simulink model "SEA_SMC_DoB"  (R2020a)
settings: Solver=FixedStepAuto  StartTime=0.0  StopTime=10.0  FixedStep=1e-4  RelTol=1e-3
undefined symbols (not defined in the file): A, B, C, D, SEA
libraries: simulink x6, cstblocks x4, cjt_library_models x1
settings Model: LastModifiedBy=Erim Can Ozcinar

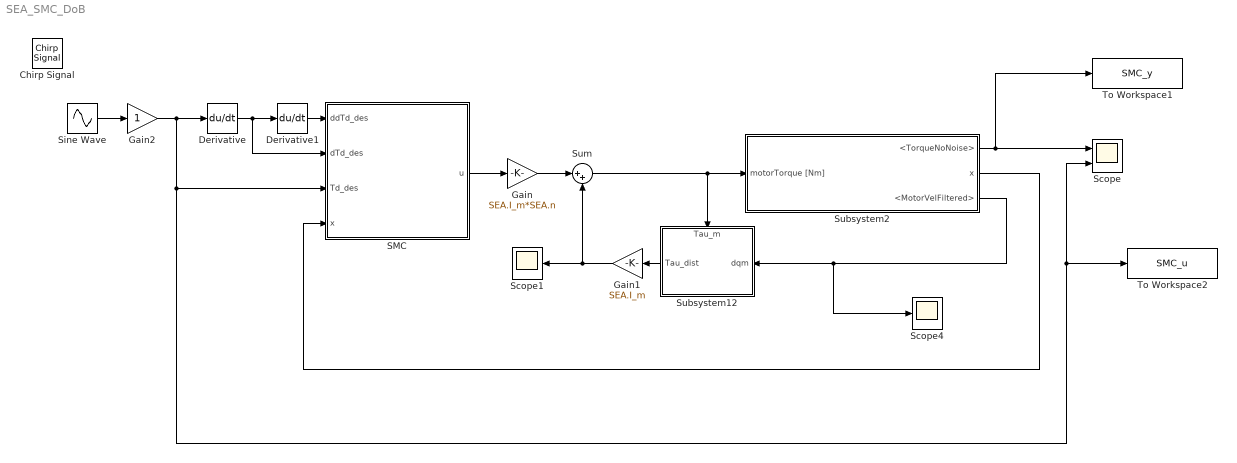
== system SEA_SMC_DoB ==
  Chirp Signal : simulink/Sources/Chirp Signal  f1=0.1  T=10  f2=25
  Derivative : Derivative
  Derivative1 : Derivative
  Gain : Gain  Gain=SEA.I_m*SEA.n
  Gain1 : Gain  Gain=SEA.I_m
  Gain2 : Gain
  SMC : MATLAB Function  TreatAsAtomicUnit=on
  Scope : Scope  NumInputPorts=2
  Scope1 : Scope
  Scope4 : Scope
  Sine Wave : Sin  SampleTime=0
  Subsystem12 : Subsystem
      settings: PortSchema="{\"entries\":[{\"content\":{\"sides\":[{\"content\":{\"connectorIds\":[\"In1\"]},\"type\":\"ConnectorPlacement.EquallySpacedRectSide\",\"uuid\":\"0907aefd-0f6e-4178-ae67-82d4302ffa8c\"},{\"content\":{\"connectorIds\":[\"Out1\"],\"side\":\"RIGHT\"},\"type\":\"ConnectorPlacement.EquallySpacedRectSide\",\"uuid\":\"771a5b93-7111-4ff8-830e-f982bc5484c0\"},{\"content\":{\"connectorIds\":[\"In2\"],\"side\":\"TOP\"},\"type\":\"ConnectorPlacement.EquallySpacedRectSide\",\"uuid\":\"5e11dad7-4fb7-439c-966f-d215f4d3795f\"}]},\"type\":\"ConnectorPlacement.EquallySpacedConnector\",\"uuid\":\"deab52ae-9dbd-41da-8fe4-7a69fd8df393\"}],\"packageUris\":[\"http://schema.mathworks.com/mf0/Connector/19700101\"],\"version\":\"1.0\"}"
  Subsystem2 : Subsystem
  Sum : Sum  Inputs=|++
  To Workspace1 : ToWorkspace  VariableName=SMC_y  SampleTime=-1
      settings: Save2DSignal=2-D array (concatenate along first dimension)
  To Workspace2 : ToWorkspace  VariableName=SMC_u  SampleTime=-1
      settings: Save2DSignal=2-D array (concatenate along first dimension)
  wires:
  Subsystem2/3(<MotorVelFiltered>) -> Scope4/1, Subsystem12/1(dqm)
  Sum/1 -> Subsystem2/1(motorTorque [Nm]), Subsystem12/2(Tau_m)
  Subsystem2/2(x) -> SMC/4(x)
  Subsystem12/1(Tau_dist) -> Gain1/1
  Gain1/1 -> Sum/2, Scope1/1
  Gain/1 -> Sum/1
  SMC/1(u) -> Gain/1
  Subsystem2/1(<TorqueNoNoise>) -> To Workspace1/1, Scope/1
  Derivative1/1 -> SMC/1(ddTd_des)
  Derivative/1 -> SMC/2(dTd_des), Derivative1/1
  Gain2/1 -> SMC/3(Td_des), Scope/2, To Workspace2/1, Derivative/1
  Sine Wave/1 -> Gain2/1

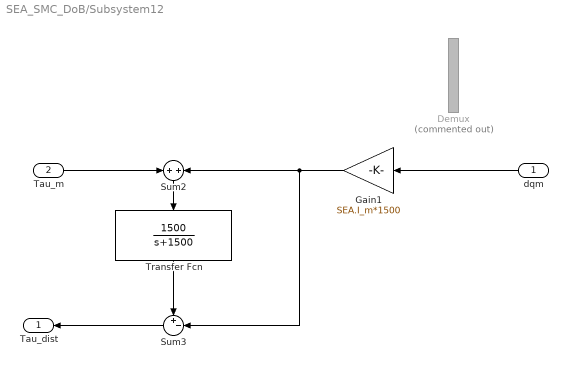
== system SEA_SMC_DoB/Subsystem12 ==
  dqm : Inport
  Tau_m : Inport  Port=2
  Demux : Demux  Commented=on  Outputs=3
  Gain1 : Gain  Gain=SEA.I_m*1500
  Sum2 : Sum  Inputs=+|+
  Sum3 : Sum  Inputs=+-|
  Transfer Fcn : TransferFcn  Numerator=[1500]  Denominator=[1 1500]
  Tau_dist : Outport
  wires:
  Gain1/1 -> Sum3/2, Sum2/2
  Sum3/1 -> Tau_dist/1
  Transfer Fcn/1 -> Sum3/1
  Tau_m/1 -> Sum2/1
  Sum2/1 -> Transfer Fcn/1
  dqm/1 -> Gain1/1

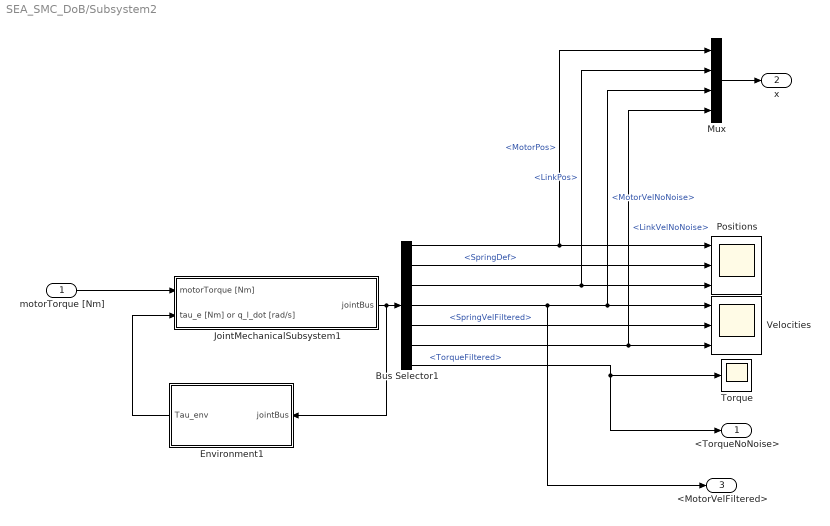
== system SEA_SMC_DoB/Subsystem2 ==
  motorTorque [Nm] : Inport
  Bus Selector1 : BusSelector  OutputSignals=MotorPos,SpringDef,LinkPos,MotorVelNoNoise,SpringVelFiltered,LinkVelNoNoise,TorqueFiltered
  Environment1 : Subsystem
  JointMechanicalSubsystem1 : Subsystem  AncestorBlock=cjt_library_models/Joint models/JointMechanicalSubsystem  mask(jointMechanicalSubsystem){jointObj=SEA, fc_vel=1000, fc_torque=1000, input_delay=0, output_delay=0, quantize=on, quantize_bits=19, input_noise_enabled=off, output_noise_enabled=off, var_u=0.000021, var_y=1e-10}
      mask prompts: jointObj "Joint Object"; fc_vel "Velocity filter cut-off frequency [Hz]"; fc_torque "Torque filter cut-off frequency [Hz]"; input_delay "Motor torque input delay (num samples of Ts)"; output_delay "Output delay (num samples of Ts)"; quantize "Quantize measurements"; quantize_bits "Quantization bits"; input_noise_enabled "Enable input noise"; output_noise_enabled "Enable measurement noise"; var_u "Input noise variance"; var_y "Measurement noise variance"
      mask help:
      | This block implements the mechanical dynamics of the actuator.
      |
      | For more information, see the > Help <.
      mask init:
      | % Get linear dynamics matrices
      | [A, B, C, D, I, R, K] = jointObj.getDynamicsMatrices();
      | 
      | % Build B matrix for nonlinear components
      | B_nonlinear = [zeros([size(B,1)-size(I,1),1]); 1./diag(I)];
      | 
      | % Get other properties
      | Ts      = jointObj.Ts;
      | Ts_elec = jointObj.Ts_elec;
      | k_b     = jointObj.k_b;
      | k_t     = jointObj.k_t;
      | n       = jointObj.n;
      | d_gl    = jointObj.d_gl;
      | 
      | % Handle MATLAB function block
      | handleMatlabFunctionBlock(gcb, jointObj);
      | 
      | % If input delay is enabled, set the flag to 1
      | input_delay_enable = 0;
      | if (input_delay > 0)
      |     input_delay_enable = 1;
      | end
      | 
      | % If noise is disabled, overwrite the given variances
      | if (input_noise_enabled == 0)
      |     var_u = 0;
      | end
      | if (output_noise_enabled == 0)
      | 	var_y = 0;
      | end
      mask Help:
      | This block implements the mechanical dynamics of the actuator. Depending on the configuration in which the joint class was built, its dynamics are given by one of the variants provided by the toolbox (see model/linear/). If provided, the linear dynamics are enhanced with nonlinear components.
      | 
      | <b>Inputs</b>
      | <b>motorTorque</b>: Electromechanical motor torque provided on the rotor. An input delay can be added to this input (e.g. due to communication delays or a very simplified representation of electrical dynamics).
      | <b>tau_e or q_l_dot</b>: External interaction torque. Depending on the selected linear dynamics model of the joint, this is either the external torque acting on the load or the imposed load velocity (for fixed-output models).
      | 
      | <b>Outputs</b>
      | <b>jointBus</b>: The various variables and their measurements, with optional delays/noise/quantisation etc. For most outputs, several instances exist. Output variables ending in "NoNoise" denote physical quantities, without noise, filtering, or delays. All other variables are affected by noise and delays (if enabled). Lastly, variables ending in "Filtered" are also low-pass filtered, with cut-off frequency set in the mask.
      | 
      | <b>An important note with regards to output variables associated with torque.</b>
      | The "Torque" and "TorqueFiltered" are computed in the way torque is usually sensed by the control system; deflection times spring constant, i.e. only the stiffness contribution is considered, as usually the internal damping of the used flexible element (parameter d_gl) is very small. Hence, TorqueFiltered is used by the toolbox controllers as well.
      | However, as noted before, "TorqueNoNoise" denotes the physical quantity. This means that it includes the torque produced by internal damping of the elastic element (parameter d_gl).
      mask Callback quantize: toggleMaskFields(gcbh, 'quantize', 'quantize_bits');
      mask Callback input_noise_enabled: toggleMaskFields(gcbh, 'input_noise_enabled', 'var_u');
      mask Callback output_noise_enabled: toggleMaskFields(gcbh, 'output_noise_enabled', 'var_y');
  Mux : Mux
  Positions : Scope  NumInputPorts=3
  Torque : Scope
  Velocities : Scope  NumInputPorts=3
  <TorqueNoNoise> : Outport
  x : Outport  Port=2
  <MotorVelFiltered> : Outport  Port=3
  wires:
  JointMechanicalSubsystem1/1(jointBus) -> Environment1/1(jointBus), Bus Selector1/1
  Mux/1 -> x/1
  Environment1/1(Tau_env) -> JointMechanicalSubsystem1/2(tau_e [Nm] or q_l_dot [rad/s])
  Bus Selector1/1 -> Mux/1, Positions/1  "<MotorPos>"
  Bus Selector1/2 -> Positions/2  "<SpringDef>"
  Bus Selector1/3 -> Mux/2, Positions/3  "<LinkPos>"
  Bus Selector1/4 -> <MotorVelFiltered>/1, Mux/3, Velocities/1  "<MotorVelNoNoise>"
  Bus Selector1/5 -> Velocities/2  "<SpringVelFiltered>"
  Bus Selector1/6 -> Mux/4, Velocities/3  "<LinkVelNoNoise>"
  Bus Selector1/7 -> <TorqueNoNoise>/1, Torque/1  "<TorqueFiltered>"
  motorTorque [Nm]/1 -> JointMechanicalSubsystem1/1(motorTorque [Nm])

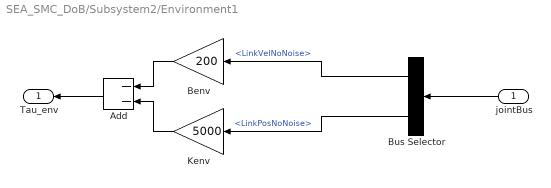
== system SEA_SMC_DoB/Subsystem2/Environment1 ==
  jointBus : Inport
  Add : Sum  Inputs=--
  Benv : Gain  Gain=200
  Bus Selector : BusSelector  OutputSignals=LinkVelNoNoise,LinkPosNoNoise
  Kenv : Gain  Gain=5000
  Tau_env : Outport
  wires:
  Kenv/1 -> Add/2
  Benv/1 -> Add/1
  Add/1 -> Tau_env/1
  Bus Selector/1 -> Benv/1  "<LinkVelNoNoise>"
  Bus Selector/2 -> Kenv/1  "<LinkPosNoNoise>"
  jointBus/1 -> Bus Selector/1

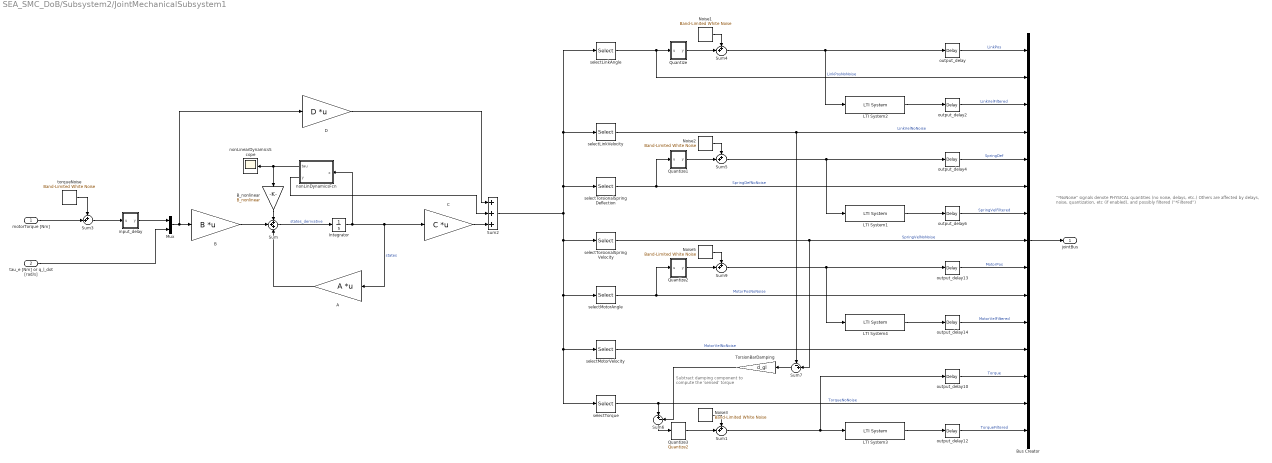
== system SEA_SMC_DoB/Subsystem2/JointMechanicalSubsystem1 ==
  note: "*NoNoise" signals denote PHYSICAL quantities (no noise, delays, etc.)
      | Others are affected by delays, noise, quantization, etc (if enabled), and possibly filtered ("*Filtered")
  note: Subtract damping component to
      | compute the 'sensed' torque
  motorTorque [Nm] : Inport
  tau_e [Nm] or q_l_dot [rad/s] : Inport  Port=2
  A : Gain  Gain=A  Multiplication=Matrix(K*u)
  B : Gain  Gain=B  Multiplication=Matrix(K*u)
  B_nonlinear : Gain  Gain=B_nonlinear
  Bus Creator : BusCreator  Inputs=15
  C : Gain  Gain=C  Multiplication=Matrix(K*u)
  D : Gain  Gain=D  Multiplication=Matrix(K*u)
  Integrator : Integrator
  LTI System1 : cstblocks/LTI System  sys=c2d(tf([2*pi*fc_vel 0], [1 2*pi*fc_vel]), Ts, 'tustin')  IC=[]
  LTI System2 : cstblocks/LTI System  sys=c2d(tf([2*pi*fc_vel 0], [1 2*pi*fc_vel]), Ts, 'tustin')  IC=[]
  LTI System3 : cstblocks/LTI System  sys=c2d(tf([2*pi*fc_torque], [1 2*pi*fc_torque]), Ts, 'tustin')  IC=[]
  LTI System4 : cstblocks/LTI System  sys=c2d(tf([2*pi*fc_vel 0], [1 2*pi*fc_vel]), Ts, 'tustin')  IC=[]
  Mux : Mux  Inputs=2
  Noise1 : simulink/Sources/Band-Limited White Noise  Cov=var_y * Ts  Ts=Ts  seed=[3846513]
  Noise2 : simulink/Sources/Band-Limited White Noise  Cov=var_y * Ts  Ts=Ts  seed=[11563454]
  Noise3 : simulink/Sources/Band-Limited White Noise  Cov=sqrt(2) * var_y * Ts % sqrt(2) accounts for subtracting two encoders  Ts=Ts  seed=[960834]
  Noise5 : simulink/Sources/Band-Limited White Noise  Cov=var_y * Ts  Ts=Ts  seed=[24326]
  Quantize : Subsystem
  Quantize1 : Subsystem
  Quantize2 : Subsystem
  Quantize3 : cjt_library_models/Joint models/JointMechanicalSubsystem/Quantize2  SystemSampleTime=-1  Latency=0  AutoFrameSizeCalculation=off
  Sum : Sum  Inputs=+++
  Sum{1,3..5,9} (5 alike) : Sum  Inputs=++|
  Sum2 : Sum  Inputs=+++
  Sum6 : Sum  Inputs=|+-
  Sum7 : Sum  Inputs=-+|
  TorsionBarDamping : Gain  Gain=d_gl
  input_delay : Subsystem
  nonLinDynamicsFcn : MATLAB Function  TreatAsAtomicUnit=on
  nonLinearDynamicsScope : Scope
  output_delay{,2,4,6,10,12..14} (8 alike) : TransportDelay  DelayTime=output_delay * jointObj.Ts
  selectLinkAngle : Selector  NumberOfDimensions=2  InputPortWidth=3  IndexOptions=Index vector (dialog),Select all  Indices=3,1  OutputSizes=1,1
  selectLinkVelocity : Selector  NumberOfDimensions=2  InputPortWidth=3  IndexOptions=Index vector (dialog),Select all  Indices=6,1  OutputSizes=1,1
  selectMotorAngle : Selector  NumberOfDimensions=2  InputPortWidth=3  IndexOptions=Index vector (dialog),Select all  Indices=1,1  OutputSizes=1,1
  selectMotorVelocity : Selector  NumberOfDimensions=2  InputPortWidth=3  IndexOptions=Index vector (dialog),Select all  Indices=4,1  OutputSizes=1,1
  selectTorque : Selector  NumberOfDimensions=2  InputPortWidth=3  IndexOptions=Index vector (dialog),Select all  Indices=7,1  OutputSizes=1,1
  selectTorsionalSpringDeflection : Selector  NumberOfDimensions=2  InputPortWidth=3  IndexOptions=Index vector (dialog),Select all  Indices=2,1  OutputSizes=1,1
  selectTorsionalSpringVelocity : Selector  NumberOfDimensions=2  InputPortWidth=3  IndexOptions=Index vector (dialog),Select all  Indices=5,1  OutputSizes=1,1
  torqueNoise : simulink/Sources/Band-Limited White Noise  Cov=var_u * Ts  Ts=Ts  seed=[2435345645]
  jointBus : Outport
  wires:
  Sum6/1 -> Quantize3/1
  Noise3/1 -> Sum1/1
  Quantize3/1 -> Sum1/2
  Sum7/1 -> TorsionBarDamping/1
  TorsionBarDamping/1 -> Sum6/2
  C/1 -> Sum2/3
  D/1 -> Sum2/1
  Quantize2/1(y) -> Sum9/2
  Quantize1/1(y) -> Sum5/2
  Quantize/1(y) -> Sum4/2
  Sum1/1 -> LTI System3/1, output_delay10/1
  LTI System3/1 -> output_delay12/1
  tau_e [Nm] or q_l_dot [rad/s]/1 -> Mux/2
  Mux/1 -> B/1, D/1
  Sum9/1 -> output_delay13/1, LTI System4/1
  output_delay14/1 -> Bus Creator/11  "MotorVelFiltered"
  output_delay13/1 -> Bus Creator/9  "MotorPos"
  LTI System4/1 -> output_delay14/1
  Noise5/1 -> Sum9/1
  output_delay12/1 -> Bus Creator/15  "TorqueFiltered"
  selectTorque/1 -> Bus Creator/14, Sum6/1  "TorqueNoNoise"
  output_delay10/1 -> Bus Creator/13  "Torque"
  selectMotorVelocity/1 -> Bus Creator/12  "MotorVelNoNoise"
  selectMotorAngle/1 -> Bus Creator/10, Quantize2/1(u)  "MotorPosNoNoise"
  selectTorsionalSpringVelocity/1 -> Sum7/2, Bus Creator/8  "SpringVelNoNoise"
  output_delay6/1 -> Bus Creator/7  "SpringVelFiltered"
  selectTorsionalSpringDeflection/1 -> Bus Creator/6, Quantize1/1(u)  "SpringDefNoNoise"
  output_delay4/1 -> Bus Creator/5  "SpringDef"
  selectLinkVelocity/1 -> Sum7/1, Bus Creator/4  "LinkVelNoNoise"
  output_delay2/1 -> Bus Creator/3  "LinkVelFiltered"
  selectLinkAngle/1 -> Bus Creator/2, Quantize/1(u)  "LinkPosNoNoise"
  output_delay/1 -> Bus Creator/1  "LinkPos"
  A/1 -> Sum/3
  B/1 -> Sum/2
  Sum2/1 -> selectTorsionalSpringDeflection/1, selectLinkVelocity/1, selectLinkAngle/1, selectMotorAngle/1, selectMotorVelocity/1, selectTorque/1, selectTorsionalSpringVelocity/1
  Integrator/1 -> A/1, C/1, nonLinDynamicsFcn/1(x)  "states"
  motorTorque [Nm]/1 -> Sum3/2
  LTI System2/1 -> output_delay2/1
  Sum/1 -> Integrator/1  "states_derivative"
  LTI System1/1 -> output_delay6/1
  Noise1/1 -> Sum4/1
  Noise2/1 -> Sum5/1
  torqueNoise/1 -> Sum3/1
  Sum4/1 -> output_delay/1, LTI System2/1
  Sum5/1 -> output_delay4/1, LTI System1/1
  Sum3/1 -> input_delay/1(u)
  input_delay/1(y) -> Mux/1
  Bus Creator/1 -> jointBus/1
  nonLinDynamicsFcn/1(tau) -> B_nonlinear/1, nonLinearDynamicsScope/1
  nonLinDynamicsFcn/2(y) -> Sum2/2
  B_nonlinear/1 -> Sum/1

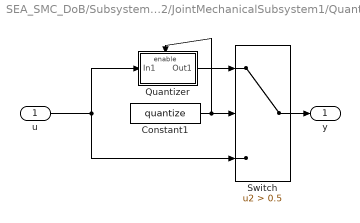
== system SEA_SMC_DoB/Subsystem2/JointMechanicalSubsystem1/Quantize ==
  u : Inport
  Constant1 : Constant  Value=quantize
  Quantizer : Subsystem
  Switch : Switch  Criteria=u2 > Threshold  Threshold=0.5
  y : Outport
  wires:
  u/1 -> Quantizer/1(In1), Switch/3
  Constant1/1 -> Quantizer/Enable, Switch/2
  Switch/1 -> y/1
  Quantizer/1(Out1) -> Switch/1

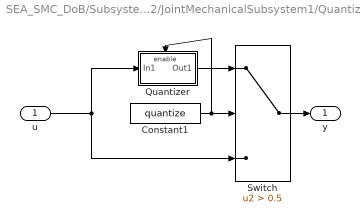
== system SEA_SMC_DoB/Subsystem2/JointMechanicalSubsystem1/Quantize1 ==
  u : Inport
  Constant1 : Constant  Value=quantize
  Quantizer : Subsystem
  Switch : Switch  Criteria=u2 > Threshold  Threshold=0.5
  y : Outport
  wires:
  u/1 -> Quantizer/1(In1), Switch/3
  Constant1/1 -> Quantizer/Enable, Switch/2
  Switch/1 -> y/1
  Quantizer/1(Out1) -> Switch/1

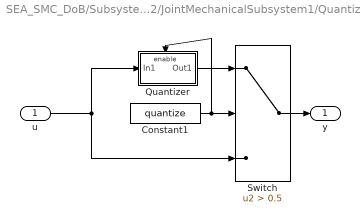
== system SEA_SMC_DoB/Subsystem2/JointMechanicalSubsystem1/Quantize2 ==
  u : Inport
  Constant1 : Constant  Value=quantize
  Quantizer : Subsystem
  Switch : Switch  Criteria=u2 > Threshold  Threshold=0.5
  y : Outport
  wires:
  u/1 -> Quantizer/1(In1), Switch/3
  Constant1/1 -> Quantizer/Enable, Switch/2
  Switch/1 -> y/1
  Quantizer/1(Out1) -> Switch/1

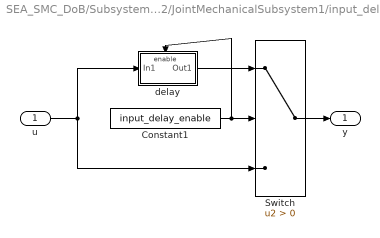
== system SEA_SMC_DoB/Subsystem2/JointMechanicalSubsystem1/input_delay ==
  u : Inport
  Constant1 : Constant  Value=input_delay_enable
  Switch : Switch  Criteria=u2 > Threshold
  delay : Subsystem
  y : Outport
  wires:
  u/1 -> delay/1(In1), Switch/3
  Constant1/1 -> Switch/2, delay/Enable
  Switch/1 -> y/1
  delay/1(Out1) -> Switch/1

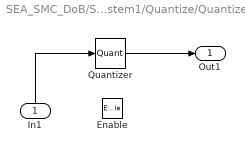
== system SEA_SMC_DoB/Subsystem2/JointMechanicalSubsystem1/Quantize/Quantizer ==
  In1 : Inport
  Enable : EnablePort
  Quantizer : Quantizer  QuantizationInterval=1/(2^quantize_bits)
  Out1 : Outport
  wires:
  In1/1 -> Quantizer/1
  Quantizer/1 -> Out1/1

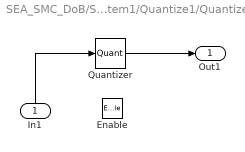
== system SEA_SMC_DoB/Subsystem2/JointMechanicalSubsystem1/Quantize1/Quantizer ==
  In1 : Inport
  Enable : EnablePort
  Quantizer : Quantizer  QuantizationInterval=1/(2^quantize_bits)
  Out1 : Outport
  wires:
  In1/1 -> Quantizer/1
  Quantizer/1 -> Out1/1

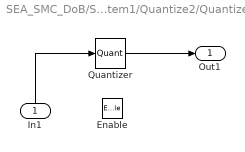
== system SEA_SMC_DoB/Subsystem2/JointMechanicalSubsystem1/Quantize2/Quantizer ==
  In1 : Inport
  Enable : EnablePort
  Quantizer : Quantizer  QuantizationInterval=1/(2^quantize_bits)
  Out1 : Outport
  wires:
  In1/1 -> Quantizer/1
  Quantizer/1 -> Out1/1

== system SEA_SMC_DoB/Subsystem2/JointMechanicalSubsystem1/input_delay/delay ==
  note: The delay value here is computed so that it is >0 when delay is DISABLED,
      | to avoid MATLAB throwing warnings unnecessarily.
  In1 : Inport
  Enable : EnablePort
  input_delay : TransportDelay  DelayTime=input_delay * jointObj.Ts + 1 - input_delay_enable  TransDelayFeedthrough=on
  Out1 : Outport
  wires:
  In1/1 -> input_delay/1
  input_delay/1 -> Out1/1

== matlab function SEA_SMC_DoB/Subsystem2/JointMechanicalSubsystem1/nonLinDynamicsFcn ==
  data: tau output; x input; y output
function [tau, y] = nonLinDynamics(x)
%#codegen

params.a_CU = 0.003900;
params.c_CU = 380.000000;
params.c_FE = 460.000000;
params.diam = 98.000000;
params.len = 166.000000;
params.m = 3.400000;
params.I_m = 0.000278;
params.I_g = 0.000000;
params.I_l = 0.070000;
params.k_g = 0.000000;
params.k_b = 5000.000000;
params.d_m = 0.001500;
params.d_g = 0.000000;
params.d_l = 0.005000;
params.d_m_n = 0.001500;
params.d_g_n = 0.000000;
params.d_l_n = 0.005000;
params.d_mg = 0.000000;
params.d_gl = 0.000000;
params.d_cm = 0.073950;
params.d_cg = 0.000000;
params.d_cl = 0.000000;
params.d_cm_n = 0.069810;
params.d_cg_n = 0.000000;
params.d_cl_n = 0.000000;
params.d_s = 0.000000;
params.v_s = 0.000000;
params.rip_types = [];
params.rip_a1 = [];
params.rip_a2 = [];
params.rip_f = [];
params.n = 100.000000;
params.k_t = 0.102000;
params.r = 0.370000;
params.x = 0.000400;
params.p = 12.000000;
params.v_0 = 48.000000;
params.i_p = 36.000000;
params.dq_p = 411.548600;
params.r_th1 = 1.637200;
params.r_th2 = 15.292500;
params.T_thw = 90.014100;
params.T_thm = 3781.168300;
params.Tmp_WMax = 155.000000;
params.Tmp_ANom = 25.000000;
params.name = 'sea_Pomegranate';
params.paramName = 'sea_param';
params.modelName = 'sea';
%params.nonlinearModelName = {'coulomb', 'viscous_asym'}; % Cell arrays are not supported for code generation.
params.electricalModelName = 'electric_dyn_2';
params.Ts = 0.001000;
params.Ts_elec = 0.000100;

[tau_1, y_1] = coulomb(params,x);
[tau_2, y_2] = viscous_asym(params,x);
tau = tau_1 +tau_2;
y = y_1 +y_2;
	end

== matlab function SEA_SMC_DoB/SMC ==
  data: ddTd_des input; dTd_des input; Td_des input; u output; x input
function u = fcn(ddTd_des, dTd_des, Td_des, x)

c = 2000;
p = 100;

Jm = (2.781e-04); % kgm^2 
Bm = (1.5e-03);   % Nms/rad
Jl = 0.07;      % kgm^2 
Bl = 0.005;     % Nms/rad
Ks = 5000;      %Nm/rad
N = 100;        % -

qm = x(1);
ql = x(2);
dqm = x(3);
dql = x(4);

qd = qm/N - ql;
dqd = dqm/N - dql;

qd_des = Td_des/Ks;
dqd_des = dTd_des/Ks;
ddqd_des = ddTd_des/Ks;

e = qd_des - qd;
de = dqd_des - dqd;

sigma = de + c*e;

u1 = Ks/(Jm*N*N) + Ks/Jl;
u2 = (Bm*Jl - Bl*Jm)/(Jm*Jl*N);

u = p*sign(sigma) + ddqd_des + u1*qd + u2*dqm + Bl*dqd/Jl + c*de ;
